simulink library "mfcm_misc_lib_v1"  (Simulink 6.1)
libraries: xbsIndex_r4 x81, mfcm_misc_lib_v1 x2, xbsCopyrightNotice_r4 x1, mfcm_mac_lib_v1 x1
settings Model: Creator=dandrews  LastModifiedBy=alexc

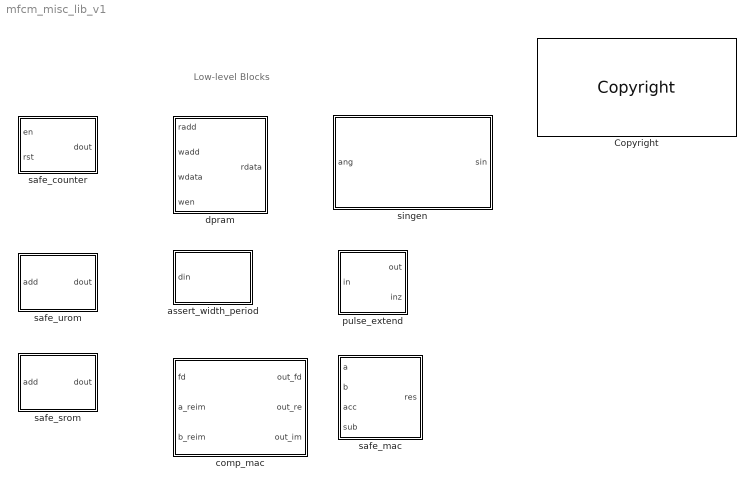
== system mfcm_misc_lib_v1 ==
  note: Low-level Blocks
  Copyright : xbsCopyrightNotice_r4/Copyright
  assert_width_period : Subsystem  mask{MIN_WIDTH=0, MAX_WIDTH=0, MIN_PERIOD=20, MAX_PERIOD=0}
      mask prompts: MIN_WIDTH "Minimum Pulse Width (0->none)"; MAX_WIDTH "Maximum Pulse Width (0->none)"; MIN_PERIOD "Minimum Pulse Period (0->none)"; MAX_PERIOD "Maximum Pulse Period (0->none)"
  comp_mac : Subsystem  mask{MULS=4, OUT_WIDTH=18, OUT_BINPT=16}
      mask prompts: MULS "Number of Multiplies"; OUT_WIDTH "Output Width"; OUT_BINPT "Output Binary Point"
      mask Display:
      | disp(sprintf('z^{%d}\n\n[z^{-(2*MULS+8)}]',-(2*MULS+8)),'texmode','on');
      | 
      | port_label('input',1,'fd');
      | port_label('input',2,'a_reim');
      | port_label('input',3,'b_reim');
      | 
      | port_label('output',1,'fd');
      | port_label('output',2,'re');
      | port_label('output',3,'im');
  dpram : Subsystem  mask{MEM_DEPTH=8192, MEM_INIT=0, MEM_MAXDEPTH=16}
      mask prompts: MEM_DEPTH "Memory Depth"; MEM_INIT "Memory Initialisation Vector"; MEM_MAXDEPTH "Maximum Distributed Memory Depth"
      mask Display:
      | disp('z^{-2}','texmode','on');
      | 
      | port_label('input',1,'radd');
      | port_label('input',2,'wadd');
      | port_label('input',3,'wdata');
      | port_label('input',4,'wen');
      | port_label('output',1,'rdata');
  pulse_extend : Subsystem  mask{WIDTH=1}
      mask prompts: WIDTH "Width of output pulse"
  safe_counter : Subsystem  mask{CNT_MAX=1}
      mask prompts: CNT_MAX "Count To Value"
      mask Display:
      | port_label('input' ,1,'en');
      | port_label('input' ,2,'rst');
      | port_label('output',1,'');
  safe_mac : Subsystem  mask{ACC_GROWTH=4, ACC_DEPTH=1}
      mask prompts: ACC_GROWTH "Accumulator Bit Width Growth"; ACC_DEPTH "Accumulator Pipeline Depth"
      mask Display:
      | disp('z^{-4}','texmode','on');
      | 
      | port_label('input',1,'a');
      | port_label('input',2,'b');
      | port_label('input',3,'acc');
      | port_label('input',4,'sub');
      | 
      | port_label('output',1,'res');
  safe_srom : Subsystem  mask{DEPTH=1, OUT_TYPE=1, OUT_WIDTH=8, OUT_BINPT=6, INIT=[1], LATENCY=1, MEM_MAXDEPTH=16}
      mask prompts: OUT_TYPE "Output Type (0->Boolean 1->Unsigned 2->Signed)"; OUT_WIDTH "Output Width"; OUT_BINPT "Output Binary Point"; INIT "Initialisation Vector"; MEM_MAXDEPTH "Maximum Distributed Memory Depth"
      mask Display:
      | disp(sprintf('z^{%d}',-LATENCY),'texmode','on');
      | port_label('input' ,1,'add');
      | port_label('output',1,'');
  safe_urom : Subsystem  mask{DEPTH=1, OUT_TYPE=1, OUT_WIDTH=8, OUT_BINPT=6, INIT=[1], LATENCY=1, MEM_MAXDEPTH=16}
      mask prompts: OUT_TYPE "Output Type (0->Boolean 1->Unsigned 2->Signed)"; OUT_WIDTH "Output Width"; OUT_BINPT "Output Binary Point"; INIT "Initialisation Vector"; MEM_MAXDEPTH "Maximum Distributed Memory Depth"
      mask Display:
      | disp(sprintf('z^{%d}',-LATENCY),'texmode','on');
      | port_label('input' ,1,'add');
      | port_label('output',1,'');
  singen : Subsystem  mask{N=8192, OUT_WIDTH=18, OUT_BINPT=17}
      mask prompts: N "Depth"; OUT_WIDTH "Output Width"; OUT_BINPT "Output Binary Point"
      mask Display:
      | disp('z^{-5}','texmode','on');
      | 
      | port_label('input',1,'ang');
      | 
      | port_label('output',1,'sin');

== system mfcm_misc_lib_v1/assert_width_period ==
  note: Wrap Mcode twice so we can use max() in MAX_CNT.
      | MCode interface does not support function calls.
  din : Inport  Port=1  LatchInput=off
  Terminator : Terminator
  x : Subsystem  mask{MIN_WIDTH=MIN_WIDTH, MAX_WIDTH=MAX_WIDTH, MIN_PERIOD=MIN_PERIOD, MAX_PERIOD=MAX_PERIOD, MAX_CNT=2^ceil(log2(max([MIN_WIDTH MAX_WIDTH MIN_PERIOD MAX_PERIOD])))}
  wires:
  x/1(fire) -> Terminator/1
  din/1 -> x/1(din)

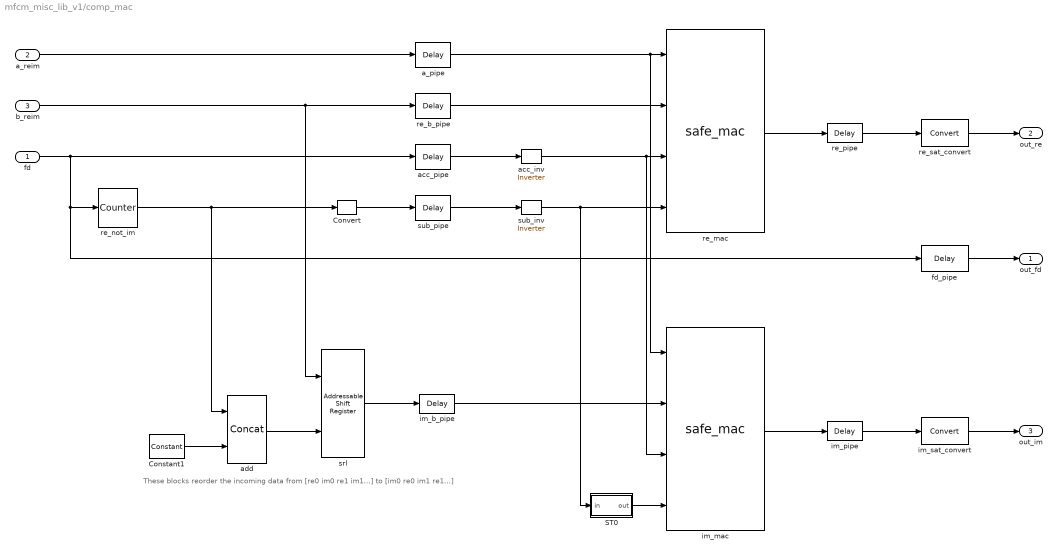
== system mfcm_misc_lib_v1/comp_mac ==
  note: These blocks reorder the incoming data from [re0 im0 re1 im1...] to [im0 re0 im1 re1...]
  fd : Inport  Port=1  LatchInput=off
  a_reim : Inport  Port=2  LatchInput=off
  b_reim : Inport  Port=3  LatchInput=off
  Constant1 : xbsIndex_r4/Constant  arith_type=Unsigned  const=0  n_bits=1  bin_pt=0  explicit_period=off  period=1  equ=P=C  opselect=C  inp2=PCIN>>17  opr=+  inp1=P  carry=CIN  dbl_ovrd=off  block_type=constant
      settings: block_version=VER_STRING_GOES_HERE
  Convert : xbsIndex_r4/Convert  arith_type=Boolean  n_bits=8  bin_pt=6  quantization=Truncate  overflow=Wrap  latency=0  dbl_ovrd=off  pipeline=off  block_type=convert
      settings: infoedit=The input is presented at the output after quantization and overflow effects.<P><P>Hardware notes: Additional hardware is used when rounding or saturation is selected and output width is less than the input width.  xl_area=[0, 0, 0, 0, 0, 0, 0]  block_version=VER_STRING_GOES_HERE
  ST0 : Subsystem
  a_pipe : xbsIndex_r4/Delay  en=off  latency=3  dbl_ovrd=off  reg_retiming=off  block_type=delay
      settings: infoedit="Delay line having  configurable length.<P><P>Hardware notes: A delay line is a chain, each link of which is an SRL16 followed by a flip-flop. If register retiming is enabled, the delay line is a chain of flip-flops."  xl_area=[0, 0, 0, 0, 0, 0, 0]  block_version=VER_STRING_GOES_HERE
  acc_inv : xbsIndex_r4/Inverter  en=off  latency=0  dbl_ovrd=off  block_type=inv
      settings: xl_area=[0, 0, 0, 0, 0, 0, 0]  block_version=VER_STRING_GOES_HERE
  acc_pipe : xbsIndex_r4/Delay  en=off  latency=3  dbl_ovrd=off  reg_retiming=off  block_type=delay
      settings: infoedit="Delay line having  configurable length.<P><P>Hardware notes: A delay line is a chain, each link of which is an SRL16 followed by a flip-flop. If register retiming is enabled, the delay line is a chain of flip-flops."  xl_area=[0, 0, 0, 0, 0, 0, 0]  block_version=VER_STRING_GOES_HERE
  add : xbsIndex_r4/Concat  num_inputs=2  dbl_ovrd=off  block_type=concat
      settings: block_version=VER_STRING_GOES_HERE
  fd_pipe : xbsIndex_r4/Delay  en=off  latency=2*MULS+3+4+2-1  dbl_ovrd=off  reg_retiming=off  block_type=delay
      settings: infoedit="Delay line having  configurable length.<P><P>Hardware notes: A delay line is a chain, each link of which is an SRL16 followed by a flip-flop. If register retiming is enabled, the delay line is a chain of flip-flops."  xl_area=[0, 0, 0, 0, 0, 0, 0]  block_version=VER_STRING_GOES_HERE
  im_b_pipe : xbsIndex_r4/Delay  en=off  latency=1  dbl_ovrd=off  reg_retiming=off  block_type=delay
      settings: infoedit="Delay line having  configurable length.<P><P>Hardware notes: A delay line is a chain, each link of which is an SRL16 followed by a flip-flop. If register retiming is enabled, the delay line is a chain of flip-flops."  xl_area=[0, 0, 0, 0, 0, 0, 0]  block_version=VER_STRING_GOES_HERE
  im_mac : mfcm_misc_lib_v1/safe_mac  ACC_GROWTH=ceil(log2(2*MULS))  ACC_DEPTH=1
  im_pipe : xbsIndex_r4/Delay  en=off  latency=1  dbl_ovrd=off  reg_retiming=off  block_type=delay
      settings: infoedit="Delay line having  configurable length.<P><P>Hardware notes: A delay line is a chain, each link of which is an SRL16 followed by a flip-flop. If register retiming is enabled, the delay line is a chain of flip-flops."  xl_area=[0, 0, 0, 0, 0, 0, 0]  block_version=VER_STRING_GOES_HERE
  im_sat_convert : xbsIndex_r4/Convert  arith_type="Signed  (2's comp)"  n_bits=OUT_WIDTH  bin_pt=OUT_BINPT  quantization=Truncate  overflow=Saturate  latency=1  dbl_ovrd=off  pipeline=off  block_type=convert
      settings: infoedit=The input is presented at the output after quantization and overflow effects.<P><P>Hardware notes: Additional hardware is used when rounding or saturation is selected and output width is less than the input width.  block_version=VER_STRING_GOES_HERE
  re_b_pipe : xbsIndex_r4/Delay  en=off  latency=3  dbl_ovrd=off  reg_retiming=off  block_type=delay
      settings: infoedit="Delay line having  configurable length.<P><P>Hardware notes: A delay line is a chain, each link of which is an SRL16 followed by a flip-flop. If register retiming is enabled, the delay line is a chain of flip-flops."  xl_area=[0, 0, 0, 0, 0, 0, 0]  block_version=VER_STRING_GOES_HERE
  re_mac : mfcm_misc_lib_v1/safe_mac  ACC_GROWTH=ceil(log2(2*MULS))  ACC_DEPTH=1
  re_not_im : xbsIndex_r4/Counter  cnt_type=Free Running  cnt_to=Inf  operation=Up  start_count=1  cnt_by_val=1  arith_type=Unsigned  n_bits=1  bin_pt=0  load_pin=off  rst=on  en=off  dbl_ovrd=off  explicit_period=off  period=1  block_type=counter
      settings: infoedit="Configurable up, down and up/down counter.<P><P>Hardware notes: Free running counters are the least expensive in hardware.  A count limited counter is implemented by combining a counter with a comparator."  xl_area=[0, 0, 0, 0, 0, 0, 0]  block_version=VER_STRING_GOES_HERE
  re_pipe : xbsIndex_r4/Delay  en=off  latency=1  dbl_ovrd=off  reg_retiming=off  block_type=delay
      settings: infoedit="Delay line having  configurable length.<P><P>Hardware notes: A delay line is a chain, each link of which is an SRL16 followed by a flip-flop. If register retiming is enabled, the delay line is a chain of flip-flops."  xl_area=[0, 0, 0, 0, 0, 0, 0]  block_version=VER_STRING_GOES_HERE
  re_sat_convert : xbsIndex_r4/Convert  arith_type="Signed  (2's comp)"  n_bits=OUT_WIDTH  bin_pt=OUT_BINPT  quantization=Truncate  overflow=Saturate  latency=1  dbl_ovrd=off  pipeline=off  block_type=convert
      settings: infoedit=The input is presented at the output after quantization and overflow effects.<P><P>Hardware notes: Additional hardware is used when rounding or saturation is selected and output width is less than the input width.  block_version=VER_STRING_GOES_HERE
  srl : xbsIndex_r4/Addressable Shift Register  infer_latency=on  depth=2  initVector=[0]  en=off  dbl_ovrd=off  use_behavioral_HDL=on  use_rpm=off  block_type=addrsr
      settings: infoedit="Delay of configurable length.  Any element in the delay line can be addressed and driven onto the output port.<P><P>Hardware notes: Implemented using SRL16s.  If a Virtex-II device is used, multiple SRLC16s are cascaded together."  xl_area=[0, 0, 0, 0, 0, 0, 0]  block_version=VER_STRING_GOES_HERE
  sub_inv : xbsIndex_r4/Inverter  en=off  latency=0  dbl_ovrd=off  block_type=inv
      settings: xl_area=[0, 0, 0, 0, 0, 0, 0]  block_version=VER_STRING_GOES_HERE
  sub_pipe : xbsIndex_r4/Delay  en=off  latency=2  dbl_ovrd=off  reg_retiming=off  block_type=delay
      settings: infoedit="Delay line having  configurable length.<P><P>Hardware notes: A delay line is a chain, each link of which is an SRL16 followed by a flip-flop. If register retiming is enabled, the delay line is a chain of flip-flops."  xl_area=[0, 0, 0, 0, 0, 0, 0]  block_version=VER_STRING_GOES_HERE
  out_fd : Outport
  out_re : Outport  Port=2
  out_im : Outport  Port=3
  wires:
  sub_pipe/1 -> sub_inv/1
  acc_pipe/1 -> acc_inv/1
  fd_pipe/1 -> out_fd/1
  a_reim/1 -> a_pipe/1
  re_mac/1 -> re_pipe/1
  b_reim/1 -> re_b_pipe/1, srl/1
  im_mac/1 -> im_pipe/1
  re_b_pipe/1 -> re_mac/2
  a_pipe/1 -> re_mac/1, im_mac/1
  fd/1 -> fd_pipe/1, re_not_im/1, acc_pipe/1
  im_sat_convert/1 -> out_im/1
  re_sat_convert/1 -> out_re/1
  ST0/1(out) -> im_mac/4
  im_b_pipe/1 -> im_mac/2
  re_not_im/1 -> add/1, Convert/1
  add/1 -> srl/2
  Constant1/1 -> add/2
  srl/1 -> im_b_pipe/1
  Convert/1 -> sub_pipe/1
  acc_inv/1 -> re_mac/3, im_mac/3
  sub_inv/1 -> ST0/1(in), re_mac/4
  re_pipe/1 -> re_sat_convert/1
  im_pipe/1 -> im_sat_convert/1

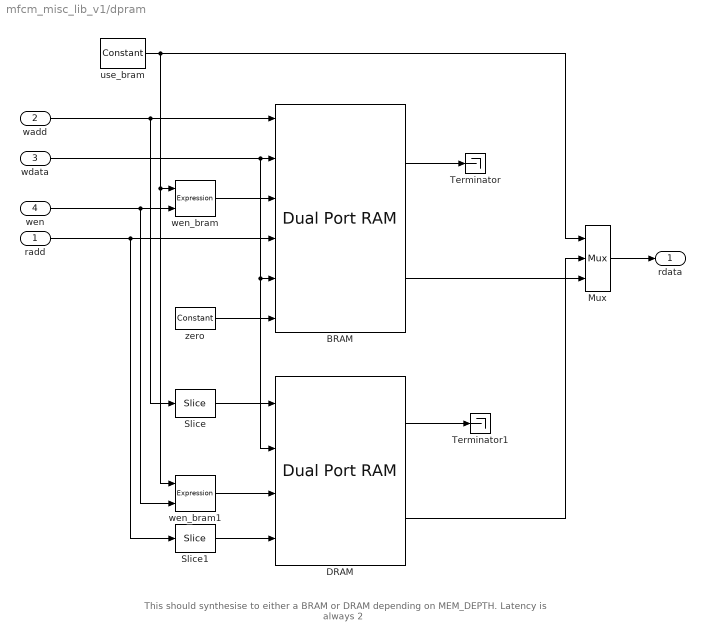
== system mfcm_misc_lib_v1/dpram ==
  note: This should synthesise to either a BRAM or DRAM depending on MEM_DEPTH.
      | Latency is always 2
  radd : Inport  Port=1  LatchInput=off
  wadd : Inport  Port=2  LatchInput=off
  wdata : Inport  Port=3  LatchInput=off
  wen : Inport  Port=4  LatchInput=off
  BRAM : xbsIndex_r4/Dual Port RAM  depth=MEM_DEPTH  initVector=MEM_INIT  distributed_mem=Block RAM  init_a=0  init_b=0  rst_a=off  rst_b=off  en_a=off  en_b=off  latency=2  write_mode_A=Read After Write  write_mode_B=Read After Write  dbl_ovrd=off  use_rpm=on  block_type=dpram
      settings: block_version=VER_STRING_GOES_HERE
  DRAM : xbsIndex_r4/Dual Port RAM  depth=min(MEM_DEPTH,MEM_MAXDEPTH)  initVector=MEM_INIT  distributed_mem=Distributed memory  init_a=0  init_b=0  rst_a=off  rst_b=off  en_a=off  en_b=off  latency=2  write_mode_A=Read After Write  write_mode_B=Read After Write  dbl_ovrd=off  use_rpm=on  block_type=dpram
      settings: block_version=VER_STRING_GOES_HERE
  Mux : xbsIndex_r4/Mux  inputs=2  en=off  latency=0  precision=Full  arith_type=Unsigned  n_bits=8  bin_pt=2  quantization=Truncate  overflow=Wrap  dbl_ovrd=off  block_type=mux
      settings: block_version=VER_STRING_GOES_HERE
  Slice : xbsIndex_r4/Slice  nbits=ceil(log2(min(MEM_DEPTH,MEM_MAXDEPTH)))  boolean_output=off  mode=Lower Bit Location + Width  bit1=0  base1=MSB of Input  bit0=0  base0=LSB of Input  dbl_ovrd=off  block_type=slice
      settings: infoedit="Extracts a given range of bits from each input sample and presents it at the output.  The output type is ordinarily unsigned with binary point at zero, but can be Boolean when the slice is one bit wide.<P><P>Hardware notes: In hardware this block costs nothing."  block_version=VER_STRING_GOES_HERE
  Slice1 : xbsIndex_r4/Slice  nbits=ceil(log2(min(MEM_DEPTH,MEM_MAXDEPTH)))  boolean_output=off  mode=Lower Bit Location + Width  bit1=0  base1=MSB of Input  bit0=0  base0=LSB of Input  dbl_ovrd=off  block_type=slice
      settings: infoedit="Extracts a given range of bits from each input sample and presents it at the output.  The output type is ordinarily unsigned with binary point at zero, but can be Boolean when the slice is one bit wide.<P><P>Hardware notes: In hardware this block costs nothing."  block_version=VER_STRING_GOES_HERE
  Terminator : Terminator
  Terminator1 : Terminator
  use_bram : xbsIndex_r4/Constant  arith_type=Boolean  const=double(MEM_DEPTH>MEM_MAXDEPTH)  n_bits=1  bin_pt=0  explicit_period=off  period=1  equ=P=C  opselect=C  inp2=PCIN>>17  opr=+  inp1=P  carry=CIN  dbl_ovrd=off  block_type=constant
      settings: block_version=VER_STRING_GOES_HERE
  wen_bram : xbsIndex_r4/Expression  expression=a & b  align_bp=on  en=off  latency=0  precision=Full  arith_type=Unsigned  n_bits=8  bin_pt=2  dbl_ovrd=off  block_type=expr
      settings: block_version=VER_STRING_GOES_HERE
  wen_bram1 : xbsIndex_r4/Expression  expression=~a & b  align_bp=on  en=off  latency=0  precision=Full  arith_type=Unsigned  n_bits=8  bin_pt=2  dbl_ovrd=off  block_type=expr
      settings: block_version=VER_STRING_GOES_HERE
  zero : xbsIndex_r4/Constant  arith_type=Boolean  const=0  n_bits=1  bin_pt=0  explicit_period=off  period=1  equ=P=C  opselect=C  inp2=PCIN>>17  opr=+  inp1=P  carry=CIN  dbl_ovrd=off  block_type=constant
      settings: block_version=VER_STRING_GOES_HERE
  rdata : Outport
  wires:
  Slice/1 -> DRAM/1
  wadd/1 -> BRAM/1, Slice/1
  wdata/1 -> BRAM/2, DRAM/2, BRAM/5
  wen_bram/1 -> BRAM/3
  use_bram/1 -> wen_bram/1, wen_bram1/1, Mux/1
  wen/1 -> wen_bram/2, wen_bram1/2
  wen_bram1/1 -> DRAM/3
  Slice1/1 -> DRAM/4
  radd/1 -> BRAM/4, Slice1/1
  zero/1 -> BRAM/6
  BRAM/1 -> Terminator/1
  DRAM/1 -> Terminator1/1
  BRAM/2 -> Mux/3
  DRAM/2 -> Mux/2
  Mux/1 -> rdata/1

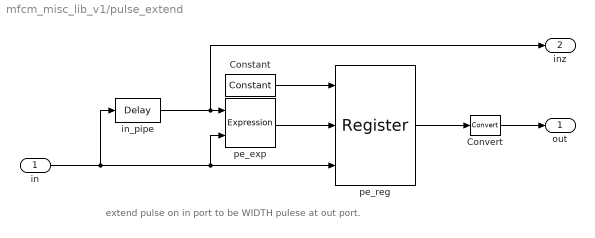
== system mfcm_misc_lib_v1/pulse_extend ==
  note: extend pulse on in port to be WIDTH pulese at out port.
  in : Inport  Port=1  LatchInput=off
  Constant : xbsIndex_r4/Constant  arith_type=Unsigned  const=1  n_bits=1  bin_pt=0  explicit_period=off  period=1  equ=P=C  opselect=C  inp2=PCIN>>17  opr=+  inp1=P  carry=CIN  dbl_ovrd=off  block_type=constant
      settings: block_version=VER_STRING_GOES_HERE
  Convert : xbsIndex_r4/Convert  arith_type=Boolean  n_bits=8  bin_pt=6  quantization=Truncate  overflow=Wrap  latency=0  dbl_ovrd=off  pipeline=off  block_type=convert
      settings: infoedit=The input is presented at the output after quantization and overflow effects.<P><P>Hardware notes: Additional hardware is used when rounding or saturation is selected and output width is less than the input width.  xl_area=[0, 0, 0, 0, 0, 0, 0]  block_version=VER_STRING_GOES_HERE
  in_pipe : xbsIndex_r4/Delay  en=off  latency=WIDTH  dbl_ovrd=off  reg_retiming=off  block_type=delay
      settings: infoedit="Delay line having  configurable length.<P><P>Hardware notes: A delay line is a chain, each link of which is an SRL16 followed by a flip-flop. If register retiming is enabled, the delay line is a chain of flip-flops."  xl_area=[0, 0, 0, 0, 0, 0, 0]  block_version=VER_STRING_GOES_HERE
  pe_exp : xbsIndex_r4/Expression  expression=a & ~b  align_bp=on  en=off  latency=0  precision=Full  arith_type=Unsigned  n_bits=8  bin_pt=2  dbl_ovrd=off  block_type=expr
      settings: xl_area=[0, 0, 0, 0, 0, 0, 0]  block_version=VER_STRING_GOES_HERE
  pe_reg : xbsIndex_r4/Register  init=0  rst=on  en=on  dbl_ovrd=off  block_type=register
      settings: xl_area=[0, 0, 0, 0, 0, 0, 0]  block_version=VER_STRING_GOES_HERE
  out : Outport
  inz : Outport  Port=2
  wires:
  in/1 -> pe_reg/3, pe_exp/2, in_pipe/1
  pe_exp/1 -> pe_reg/2
  in_pipe/1 -> pe_exp/1, inz/1
  Constant/1 -> pe_reg/1
  pe_reg/1 -> Convert/1
  Convert/1 -> out/1

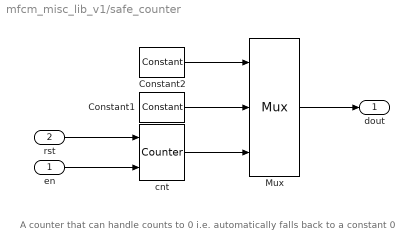
== system mfcm_misc_lib_v1/safe_counter ==
  note: A counter that can handle counts to 0
      | i.e. automatically falls back to a constant 0
  en : Inport  Port=1  LatchInput=off
  rst : Inport  Port=2  LatchInput=off
  Constant1 : xbsIndex_r4/Constant  arith_type=Unsigned  const=0  n_bits=1  bin_pt=0  explicit_period=off  period=1  equ=P=C  opselect=C  inp2=PCIN>>17  opr=+  inp1=P  carry=CIN  dbl_ovrd=off  block_type=constant
      settings: block_version=VER_STRING_GOES_HERE
  Constant2 : xbsIndex_r4/Constant  arith_type=Boolean  const=double(CNT_MAX>0)  n_bits=1  bin_pt=0  explicit_period=off  period=1  equ=P=C  opselect=C  inp2=PCIN>>17  opr=+  inp1=P  carry=CIN  dbl_ovrd=off  block_type=constant
      settings: block_version=VER_STRING_GOES_HERE
  Mux : xbsIndex_r4/Mux  inputs=2  en=off  latency=0  precision=Full  arith_type="Signed  (2's comp)"  n_bits=8  bin_pt=2  quantization=Truncate  overflow=Wrap  dbl_ovrd=off  block_type=mux
      settings: xl_area=[0, 0, 0, 0, 0, 0, 0]  block_version=VER_STRING_GOES_HERE
  cnt : xbsIndex_r4/Counter  cnt_type=Count Limited  cnt_to=max(CNT_MAX,1)  operation=Up  start_count=0  cnt_by_val=1  arith_type=Unsigned  n_bits=max(ceil(log2(CNT_MAX+1)),1)  bin_pt=0  load_pin=off  rst=on  en=on  dbl_ovrd=off  explicit_period=off  period=1  block_type=counter
      settings: infoedit="Configurable up, down and up/down counter.<P><P>Hardware notes: Free running counters are the least expensive in hardware.  A count limited counter is implemented by combining a counter with a comparator."  block_version=VER_STRING_GOES_HERE
  dout : Outport
  wires:
  Constant2/1 -> Mux/1
  Constant1/1 -> Mux/2
  cnt/1 -> Mux/3
  Mux/1 -> dout/1
  rst/1 -> cnt/1
  en/1 -> cnt/2

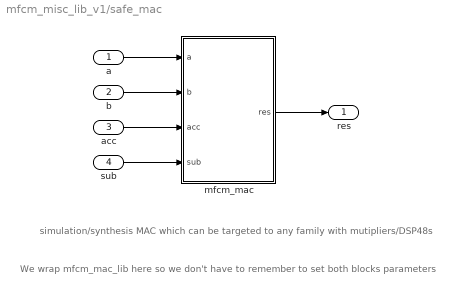
== system mfcm_misc_lib_v1/safe_mac ==
  note: simulation/synthesis MAC which can be targeted
      | to any family with mutipliers/DSP48s
  note: We wrap mfcm_mac_lib here so we don't have to
      | remember to set both blocks parameters
  a : Inport  Port=1  LatchInput=off
  b : Inport  Port=2  LatchInput=off
  acc : Inport  Port=3  LatchInput=off
  sub : Inport  Port=4  LatchInput=off
  mfcm_mac : Subsystem  Tag=configX  BlockChoice=mfcm_mac_sim
      link override mfcm_mac_sim: ACC_GROWTH=ACC_GROWTH  ACC_DEPTH=ACC_DEPTH
      link override mfcm_mac_syn: ACC_GROWTH=ACC_GROWTH  ACC_DEPTH=ACC_DEPTH
      settings: AttributesFormatString=%<BlockChoice>  TemplateBlock=mfcm_mac_lib_v1/mfcm_mac  MemberBlocks=mfcm_mac_sim,mfcm_mac_syn
  res : Outport
  wires:
  a/1 -> mfcm_mac/1(a)
  b/1 -> mfcm_mac/2(b)
  mfcm_mac/1(res) -> res/1
  acc/1 -> mfcm_mac/3(acc)
  sub/1 -> mfcm_mac/4(sub)

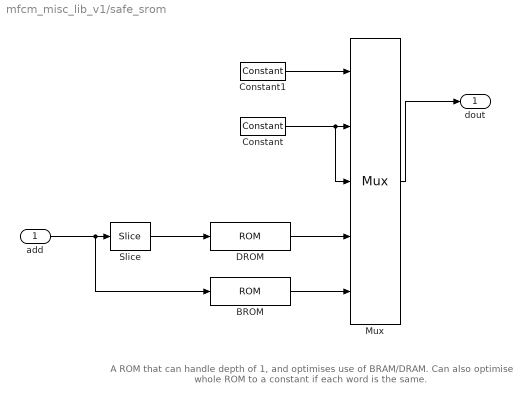
== system mfcm_misc_lib_v1/safe_srom ==
  note: A ROM that can handle depth of 1, and optimises use of BRAM/DRAM.
      | Can also optimise whole ROM to a constant if each word is the same.
  add : Inport  Port=1  LatchInput=off
  BROM : xbsIndex_r4/ROM  depth=max(DEPTH,2)  initVector=INIT  distributed_mem=Distributed memory  rst=off  init_reg=0  en=off  latency=LATENCY  arith_type="Signed  (2's comp)"  n_bits=OUT_WIDTH  bin_pt=OUT_BINPT  dbl_ovrd=off  use_rpm=off  block_type=sprom
      settings: xl_area=[0, 0, 0, 0, 0, 0, 0]  block_version=VER_STRING_GOES_HERE
  Constant : xbsIndex_r4/Constant  arith_type=Signed (2's comp)  const=min(INIT)  n_bits=OUT_WIDTH  bin_pt=OUT_BINPT  explicit_period=off  period=1  equ=P=C  opselect=C  inp2=PCIN>>17  opr=+  inp1=P  carry=CIN  dbl_ovrd=off  block_type=constant
      settings: block_version=VER_STRING_GOES_HERE
  Constant1 : xbsIndex_r4/Constant  arith_type=Unsigned  const=2*double(min(INIT)~=max(INIT))+double(DEPTH>MEM_MAXDEPTH)  n_bits=2  bin_pt=0  explicit_period=off  period=1  equ=P=C  opselect=C  inp2=PCIN>>17  opr=+  inp1=P  carry=CIN  dbl_ovrd=off  block_type=constant
      settings: block_version=VER_STRING_GOES_HERE
  DROM : xbsIndex_r4/ROM  depth=min(max(DEPTH,2),MEM_MAXDEPTH)  initVector=INIT  distributed_mem=Distributed memory  rst=off  init_reg=0  en=off  latency=LATENCY  arith_type="Signed  (2's comp)"  n_bits=OUT_WIDTH  bin_pt=OUT_BINPT  dbl_ovrd=off  use_rpm=off  block_type=sprom
      settings: xl_area=[0, 0, 0, 0, 0, 0, 0]  block_version=VER_STRING_GOES_HERE
  Mux : xbsIndex_r4/Mux  inputs=4  en=off  latency=0  precision=Full  arith_type="Signed  (2's comp)"  n_bits=8  bin_pt=2  quantization=Truncate  overflow=Wrap  dbl_ovrd=off  block_type=mux
      settings: xl_area=[0, 0, 0, 0, 0, 0, 0]  block_version=VER_STRING_GOES_HERE
  Slice : xbsIndex_r4/Slice  nbits=ceil(log2(min(max(DEPTH,2),MEM_MAXDEPTH)))  boolean_output=off  mode=Lower Bit Location + Width  bit1=0  base1=MSB of Input  bit0=0  base0=LSB of Input  dbl_ovrd=off  block_type=slice
      settings: infoedit="Extracts a given range of bits from each input sample and presents it at the output.  The output type is ordinarily unsigned with binary point at zero, but can be Boolean when the slice is one bit wide.<P><P>Hardware notes: In hardware this block costs nothing."  block_version=VER_STRING_GOES_HERE
  dout : Outport
  wires:
  Slice/1 -> DROM/1
  BROM/1 -> Mux/5
  DROM/1 -> Mux/4
  Constant/1 -> Mux/3, Mux/2
  add/1 -> BROM/1, Slice/1
  Mux/1 -> dout/1
  Constant1/1 -> Mux/1

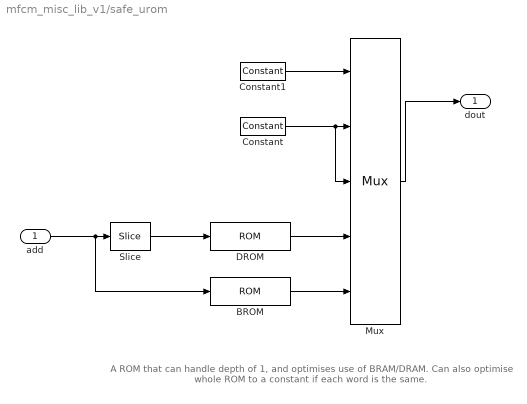
== system mfcm_misc_lib_v1/safe_urom ==
  note: A ROM that can handle depth of 1, and optimises use of BRAM/DRAM.
      | Can also optimise whole ROM to a constant if each word is the same.
  add : Inport  Port=1  LatchInput=off
  BROM : xbsIndex_r4/ROM  depth=max(DEPTH,2)  initVector=INIT  distributed_mem=Distributed memory  rst=off  init_reg=0  en=off  latency=LATENCY  arith_type=Unsigned  n_bits=OUT_WIDTH  bin_pt=OUT_BINPT  dbl_ovrd=off  use_rpm=off  block_type=sprom
      settings: xl_area=[0, 0, 0, 0, 0, 0, 0]  block_version=VER_STRING_GOES_HERE
  Constant : xbsIndex_r4/Constant  arith_type=Unsigned  const=min(INIT)  n_bits=OUT_WIDTH  bin_pt=OUT_BINPT  explicit_period=off  period=1  equ=P=C  opselect=C  inp2=PCIN>>17  opr=+  inp1=P  carry=CIN  dbl_ovrd=off  block_type=constant
      settings: block_version=VER_STRING_GOES_HERE
  Constant1 : xbsIndex_r4/Constant  arith_type=Unsigned  const=2*double(min(INIT)~=max(INIT))+double(DEPTH>MEM_MAXDEPTH)  n_bits=2  bin_pt=0  explicit_period=off  period=1  equ=P=C  opselect=C  inp2=PCIN>>17  opr=+  inp1=P  carry=CIN  dbl_ovrd=off  block_type=constant
      settings: block_version=VER_STRING_GOES_HERE
  DROM : xbsIndex_r4/ROM  depth=min(max(DEPTH,2),MEM_MAXDEPTH)  initVector=INIT  distributed_mem=Distributed memory  rst=off  init_reg=0  en=off  latency=LATENCY  arith_type=Unsigned  n_bits=OUT_WIDTH  bin_pt=OUT_BINPT  dbl_ovrd=off  use_rpm=off  block_type=sprom
      settings: xl_area=[0, 0, 0, 0, 0, 0, 0]  block_version=VER_STRING_GOES_HERE
  Mux : xbsIndex_r4/Mux  inputs=4  en=off  latency=0  precision=Full  arith_type="Signed  (2's comp)"  n_bits=8  bin_pt=2  quantization=Truncate  overflow=Wrap  dbl_ovrd=off  block_type=mux
      settings: xl_area=[0, 0, 0, 0, 0, 0, 0]  block_version=VER_STRING_GOES_HERE
  Slice : xbsIndex_r4/Slice  nbits=ceil(log2(min(max(DEPTH,2),MEM_MAXDEPTH)))  boolean_output=off  mode=Lower Bit Location + Width  bit1=0  base1=MSB of Input  bit0=0  base0=LSB of Input  dbl_ovrd=off  block_type=slice
      settings: infoedit="Extracts a given range of bits from each input sample and presents it at the output.  The output type is ordinarily unsigned with binary point at zero, but can be Boolean when the slice is one bit wide.<P><P>Hardware notes: In hardware this block costs nothing."  block_version=VER_STRING_GOES_HERE
  dout : Outport
  wires:
  Constant1/1 -> Mux/1
  Mux/1 -> dout/1
  add/1 -> Slice/1, BROM/1
  Constant/1 -> Mux/2, Mux/3
  DROM/1 -> Mux/4
  BROM/1 -> Mux/5
  Slice/1 -> DROM/1

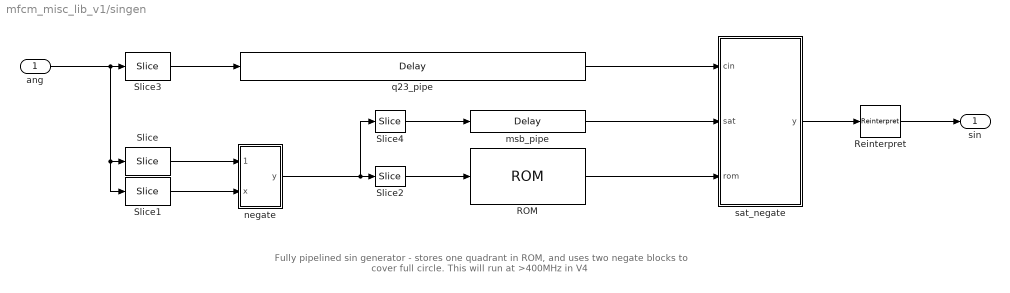
== system mfcm_misc_lib_v1/singen ==
  note: Fully pipelined sin generator - stores one quadrant in ROM, and uses two negate blocks to cover full circle.
      | This will run at >400MHz in V4
  ang : Inport  Port=1  LatchInput=off
  ROM : xbsIndex_r4/ROM  depth=N/4  initVector=min(round(sin([0:N/4-1]*2*pi/N)*2^OUT_BINPT),(2^OUT_WIDTH-1)-1)+floor(round(sin([0:N/4-1]*2*pi/N)*2^OUT_BINPT)/2^OUT_BINPT)*2^(OUT_WIDTH-1)*double((OUT_WIDTH-OUT_BINPT)<=1)  distributed_mem=Block RAM  rst=off  init_reg=0  en=off  latency=2  arith_type=Unsigned  n_bits=OUT_WIDTH  bin_pt=0  dbl_ovrd=off  use_rpm=off  block_type=sprom
      settings: xl_area=[0, 0, 0, 0, 0, 0, 0]  block_version=VER_STRING_GOES_HERE
  Reinterpret : xbsIndex_r4/Reinterpret  force_arith_type=on  arith_type="Signed  (2's comp)"  force_bin_pt=on  bin_pt=OUT_BINPT  block_type=cast
      settings: infoedit="Changes type of samples without altering their binary representation.<P><P>Hardware notes: In hardware this block costs nothing.<P><P>Example:  Suppose the input is 6 bits wide, signed, with 2 fractional bits, and the output is forced to unsigned with 0 fractional bits.  Then an input of -2.0 (1110.00 in binary 2's complement) becomes an output of 56 (111000 in binary)."  block_version=VER_STRING_GOES_HERE
  Slice : xbsIndex_r4/Slice  nbits=1  boolean_output=on  mode=Upper Bit Location + Width  bit1=-1  base1=MSB of Input  bit0=0  base0=LSB of Input  dbl_ovrd=off  block_type=slice
      settings: infoedit="Extracts a given range of bits from each input sample and presents it at the output.  The output type is ordinarily unsigned with binary point at zero, but can be Boolean when the slice is one bit wide.<P><P>Hardware notes: In hardware this block costs nothing."  block_version=VER_STRING_GOES_HERE
  Slice1 : xbsIndex_r4/Slice  nbits=log2(N)-2  boolean_output=off  mode=Lower Bit Location + Width  bit1=0  base1=MSB of Input  bit0=0  base0=LSB of Input  dbl_ovrd=off  block_type=slice
      settings: infoedit="Extracts a given range of bits from each input sample and presents it at the output.  The output type is ordinarily unsigned with binary point at zero, but can be Boolean when the slice is one bit wide.<P><P>Hardware notes: In hardware this block costs nothing."  block_version=VER_STRING_GOES_HERE
  Slice2 : xbsIndex_r4/Slice  nbits=log2(N)-2  boolean_output=off  mode=Lower Bit Location + Width  bit1=-1  base1=MSB of Input  bit0=0  base0=LSB of Input  dbl_ovrd=off  block_type=slice
      settings: infoedit="Extracts a given range of bits from each input sample and presents it at the output.  The output type is ordinarily unsigned with binary point at zero, but can be Boolean when the slice is one bit wide.<P><P>Hardware notes: In hardware this block costs nothing."  block_version=VER_STRING_GOES_HERE
  Slice3 : xbsIndex_r4/Slice  nbits=1  boolean_output=on  mode=Upper Bit Location + Width  bit1=0  base1=MSB of Input  bit0=0  base0=LSB of Input  dbl_ovrd=off  block_type=slice
      settings: infoedit="Extracts a given range of bits from each input sample and presents it at the output.  The output type is ordinarily unsigned with binary point at zero, but can be Boolean when the slice is one bit wide.<P><P>Hardware notes: In hardware this block costs nothing."  block_version=VER_STRING_GOES_HERE
  Slice4 : xbsIndex_r4/Slice  nbits=1  boolean_output=on  mode=Upper Bit Location + Width  bit1=0  base1=MSB of Input  bit0=0  base0=LSB of Input  dbl_ovrd=off  block_type=slice
      settings: infoedit="Extracts a given range of bits from each input sample and presents it at the output.  The output type is ordinarily unsigned with binary point at zero, but can be Boolean when the slice is one bit wide.<P><P>Hardware notes: In hardware this block costs nothing."  block_version=VER_STRING_GOES_HERE
  msb_pipe : xbsIndex_r4/Delay  en=off  latency=2  dbl_ovrd=off  reg_retiming=off  block_type=delay
      settings: infoedit="Delay line having  configurable length.<P><P>Hardware notes: A delay line is a chain, each link of which is an SRL16 followed by a flip-flop. If register retiming is enabled, the delay line is a chain of flip-flops."  xl_area=[0, 0, 0, 0, 0, 0, 0]  block_version=VER_STRING_GOES_HERE
  negate : Subsystem
  q23_pipe : xbsIndex_r4/Delay  en=off  latency=3  dbl_ovrd=off  reg_retiming=off  block_type=delay
      settings: infoedit="Delay line having  configurable length.<P><P>Hardware notes: A delay line is a chain, each link of which is an SRL16 followed by a flip-flop. If register retiming is enabled, the delay line is a chain of flip-flops."  xl_area=[0, 0, 0, 0, 0, 0, 0]  block_version=VER_STRING_GOES_HERE
  sat_negate : Subsystem
  sin : Outport
  wires:
  Slice3/1 -> q23_pipe/1
  ROM/1 -> sat_negate/3(rom)
  ang/1 -> Slice3/1, Slice1/1, Slice/1
  negate/1(y) -> Slice4/1, Slice2/1
  Slice2/1 -> ROM/1
  Slice4/1 -> msb_pipe/1
  msb_pipe/1 -> sat_negate/2(sat)
  sat_negate/1(y) -> Reinterpret/1
  Reinterpret/1 -> sin/1
  Slice/1 -> negate/1(negate)
  Slice1/1 -> negate/2(x)
  q23_pipe/1 -> sat_negate/1(cin)

== system mfcm_misc_lib_v1/assert_width_period/x ==
  din : Inport  Port=1  LatchInput=off
  x : xbsIndex_r4/MCode  mfname=mfcm_assert_width_period  explicit_period=off  period=1  dbl_ovrd=off  enable_debug=off  block_type=mcode  suppress_output=1  defparams={'MIN_WIDTH',MIN_WIDTH,'MAX_WIDTH',MAX_WIDTH,'MIN_PERIOD',MIN_PERIOD,'MAX_PERIOD',MAX_PERIOD,'MAX_CNT',16777215}  hide_port_list={}
      settings: block_version=8.1
  fire : Outport
  wires:
  din/1 -> x/1
  x/1 -> fire/1

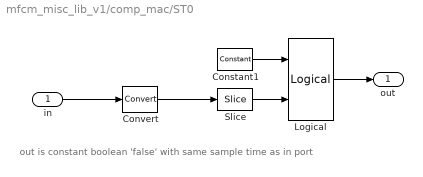
== system mfcm_misc_lib_v1/comp_mac/ST0 ==
  note: out is constant boolean 'false' with same
      | sample time as in port
  in : Inport  Port=1  LatchInput=off
  Constant1 : xbsIndex_r4/Constant  arith_type=Boolean  const=0  n_bits=1  bin_pt=0  explicit_period=off  period=1  equ=P=C  opselect=C  inp2=PCIN>>17  opr=+  inp1=P  carry=CIN  dbl_ovrd=off  block_type=constant
      settings: block_version=VER_STRING_GOES_HERE
  Convert : xbsIndex_r4/Convert  arith_type=Unsigned  n_bits=1  bin_pt=0  quantization=Truncate  overflow=Wrap  latency=0  dbl_ovrd=off  pipeline=off  block_type=convert
      settings: infoedit=The input is presented at the output after quantization and overflow effects.<P><P>Hardware notes: Additional hardware is used when rounding or saturation is selected and output width is less than the input width.  xl_area=[0, 0, 0, 0, 0, 0, 0]  block_version=VER_STRING_GOES_HERE
  Logical : xbsIndex_r4/Logical  logical_function=AND  inputs=2  en=off  latency=0  precision=Full  arith_type=Unsigned  n_bits=8  bin_pt=2  align_bp=on  dbl_ovrd=off  block_type=logical
      settings: xl_area=[0, 0, 0, 0, 0, 0, 0]  block_version=VER_STRING_GOES_HERE
  Slice : xbsIndex_r4/Slice  nbits=1  boolean_output=on  mode=Lower Bit Location + Width  bit1=0  base1=MSB of Input  bit0=0  base0=LSB of Input  dbl_ovrd=off  block_type=slice
      settings: infoedit="Extracts a given range of bits from each input sample and presents it at the output.  The output type is ordinarily unsigned with binary point at zero, but can be Boolean when the slice is one bit wide.<P><P>Hardware notes: In hardware this block costs nothing."  block_version=VER_STRING_GOES_HERE
  out : Outport
  wires:
  Constant1/1 -> Logical/1
  Convert/1 -> Slice/1
  in/1 -> Convert/1
  Logical/1 -> out/1
  Slice/1 -> Logical/2

== system mfcm_misc_lib_v1/safe_mac/mfcm_mac ==
  a : Inport  Port=1  LatchInput=off
  b : Inport  Port=2  LatchInput=off
  acc : Inport  Port=3  LatchInput=off
  sub : Inport  Port=4  LatchInput=off
  mfcm_mac_sim : mfcm_mac_lib_v1/mfcm_mac_sim  ACC_GROWTH=ACC_GROWTH  ACC_DEPTH=ACC_DEPTH
  res : Outport
  wires:
  a/1 -> mfcm_mac_sim/1
  b/1 -> mfcm_mac_sim/2
  acc/1 -> mfcm_mac_sim/3
  sub/1 -> mfcm_mac_sim/4
  mfcm_mac_sim/1 -> res/1

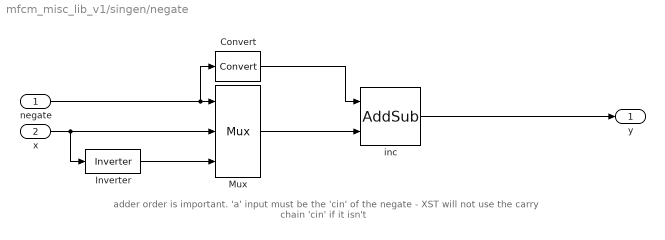
== system mfcm_misc_lib_v1/singen/negate ==
  note: adder order is important. 'a' input must be the 'cin' of the negate - XST will not use the carry chain 'cin' if it isn't
  negate : Inport  Port=1  LatchInput=off
  x : Inport  Port=2  LatchInput=off
  Convert : xbsIndex_r4/Convert  arith_type=Unsigned  n_bits=1  bin_pt=0  quantization=Truncate  overflow=Wrap  latency=0  dbl_ovrd=off  pipeline=off  block_type=convert
      settings: infoedit=The input is presented at the output after quantization and overflow effects.<P><P>Hardware notes: Additional hardware is used when rounding or saturation is selected and output width is less than the input width.  block_version=VER_STRING_GOES_HERE
  Inverter : xbsIndex_r4/Inverter  en=off  latency=0  dbl_ovrd=off  block_type=inv
      settings: block_version=VER_STRING_GOES_HERE
  Mux : xbsIndex_r4/Mux  inputs=2  en=off  latency=0  precision=Full  arith_type=Unsigned  n_bits=8  bin_pt=2  quantization=Truncate  overflow=Wrap  dbl_ovrd=off  block_type=mux
      settings: block_version=VER_STRING_GOES_HERE
  inc : xbsIndex_r4/AddSub  mode=Addition  use_carryin=off  use_carryout=off  en=off  latency=1  precision=Full  arith_type=Unsigned  n_bits=1  bin_pt=0  quantization=Truncate  overflow=Wrap  dbl_ovrd=off  use_behavioral_HDL=on  pipelined=off  use_rpm=on  block_type=addsub
      settings: block_version=VER_STRING_GOES_HERE
  y : Outport
  wires:
  Inverter/1 -> Mux/3
  x/1 -> Inverter/1, Mux/2
  negate/1 -> Mux/1, Convert/1
  inc/1 -> y/1
  Convert/1 -> inc/1
  Mux/1 -> inc/2

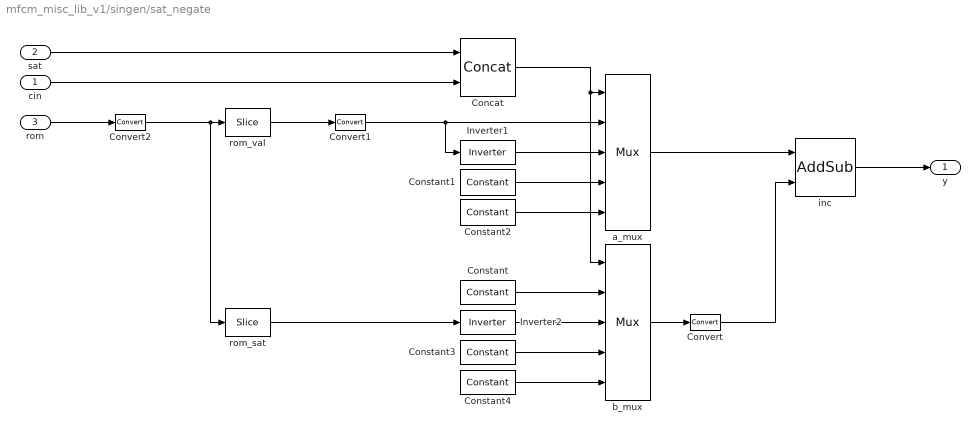
== system mfcm_misc_lib_v1/singen/sat_negate ==
  cin : Inport  Port=1  LatchInput=off
  sat : Inport  Port=2  LatchInput=off
  rom : Inport  Port=3  LatchInput=off
  Concat : xbsIndex_r4/Concat  num_inputs=2  dbl_ovrd=off  block_type=concat
      settings: block_version=VER_STRING_GOES_HERE
  Constant : xbsIndex_r4/Constant  arith_type=Boolean  const=0  n_bits=1  bin_pt=0  explicit_period=off  period=1  equ=P=C  opselect=C  inp2=PCIN>>17  opr=+  inp1=P  carry=CIN  dbl_ovrd=off  block_type=constant
      settings: block_version=VER_STRING_GOES_HERE
  Constant1 : xbsIndex_r4/Constant  arith_type=Unsigned  const=min(2^OUT_BINPT,2^(OUT_WIDTH-1)-1)  n_bits=OUT_WIDTH  bin_pt=0  explicit_period=off  period=1  equ=P=C  opselect=C  inp2=PCIN>>17  opr=+  inp1=P  carry=CIN  dbl_ovrd=off  block_type=constant
      settings: block_version=VER_STRING_GOES_HERE
  Constant2 : xbsIndex_r4/Constant  arith_type=Unsigned  const=2^OUT_WIDTH+max(-2^OUT_BINPT,-2^(OUT_WIDTH-1))-1  n_bits=OUT_WIDTH  bin_pt=0  explicit_period=off  period=1  equ=P=C  opselect=C  inp2=PCIN>>17  opr=+  inp1=P  carry=CIN  dbl_ovrd=off  block_type=constant
      settings: block_version=VER_STRING_GOES_HERE
  Constant3 : xbsIndex_r4/Constant  arith_type=Boolean  const=0  n_bits=1  bin_pt=0  explicit_period=off  period=1  equ=P=C  opselect=C  inp2=PCIN>>17  opr=+  inp1=P  carry=CIN  dbl_ovrd=off  block_type=constant
      settings: block_version=VER_STRING_GOES_HERE
  Constant4 : xbsIndex_r4/Constant  arith_type=Boolean  const=1  n_bits=1  bin_pt=0  explicit_period=off  period=1  equ=P=C  opselect=C  inp2=PCIN>>17  opr=+  inp1=P  carry=CIN  dbl_ovrd=off  block_type=constant
      settings: block_version=VER_STRING_GOES_HERE
  Convert : xbsIndex_r4/Convert  arith_type=Unsigned  n_bits=1  bin_pt=0  quantization=Truncate  overflow=Wrap  latency=0  dbl_ovrd=off  pipeline=off  block_type=convert
      settings: infoedit=The input is presented at the output after quantization and overflow effects.<P><P>Hardware notes: Additional hardware is used when rounding or saturation is selected and output width is less than the input width.  block_version=VER_STRING_GOES_HERE
  Convert1 : xbsIndex_r4/Convert  arith_type=Unsigned  n_bits=OUT_WIDTH  bin_pt=0  quantization=Truncate  overflow=Wrap  latency=0  dbl_ovrd=off  pipeline=off  block_type=convert
      settings: infoedit=The input is presented at the output after quantization and overflow effects.<P><P>Hardware notes: Additional hardware is used when rounding or saturation is selected and output width is less than the input width.  block_version=VER_STRING_GOES_HERE
  Convert2 : xbsIndex_r4/Convert  arith_type=Unsigned  n_bits=OUT_WIDTH+double((OUT_WIDTH-OUT_BINPT)>1)  bin_pt=0  quantization=Truncate  overflow=Wrap  latency=0  dbl_ovrd=off  pipeline=off  block_type=convert
      settings: infoedit=The input is presented at the output after quantization and overflow effects.<P><P>Hardware notes: Additional hardware is used when rounding or saturation is selected and output width is less than the input width.  block_version=VER_STRING_GOES_HERE
  Inverter1 : xbsIndex_r4/Inverter  en=off  latency=0  dbl_ovrd=off  block_type=inv
      settings: block_version=VER_STRING_GOES_HERE
  Inverter2 : xbsIndex_r4/Inverter  en=off  latency=0  dbl_ovrd=off  block_type=inv
      settings: block_version=VER_STRING_GOES_HERE
  a_mux : xbsIndex_r4/Mux  inputs=4  en=off  latency=1  precision=Full  arith_type=Unsigned  n_bits=8  bin_pt=2  quantization=Truncate  overflow=Wrap  dbl_ovrd=off  block_type=mux
      settings: block_version=VER_STRING_GOES_HERE
  b_mux : xbsIndex_r4/Mux  inputs=4  en=off  latency=1  precision=Full  arith_type=Unsigned  n_bits=8  bin_pt=2  quantization=Truncate  overflow=Wrap  dbl_ovrd=off  block_type=mux
      settings: block_version=VER_STRING_GOES_HERE
  inc : xbsIndex_r4/AddSub  mode=Addition  use_carryin=off  use_carryout=off  en=off  latency=1  precision=User Defined  arith_type=Unsigned  n_bits=OUT_WIDTH  bin_pt=0  quantization=Truncate  overflow=Wrap  dbl_ovrd=off  use_behavioral_HDL=on  pipelined=off  use_rpm=on  block_type=addsub
      settings: block_version=VER_STRING_GOES_HERE
  rom_sat : xbsIndex_r4/Slice  nbits=1  boolean_output=on  mode=Upper Bit Location + Width  bit1=0  base1=MSB of Input  bit0=0  base0=LSB of Input  dbl_ovrd=off  block_type=slice
      settings: infoedit="Extracts a given range of bits from each input sample and presents it at the output.  The output type is ordinarily unsigned with binary point at zero, but can be Boolean when the slice is one bit wide.<P><P>Hardware notes: In hardware this block costs nothing."  block_version=VER_STRING_GOES_HERE
  rom_val : xbsIndex_r4/Slice  nbits=OUT_WIDTH-double((OUT_WIDTH-OUT_BINPT)<=1)  boolean_output=off  mode=Lower Bit Location + Width  bit1=0  base1=MSB of Input  bit0=0  base0=LSB of Input  dbl_ovrd=off  block_type=slice
      settings: infoedit="Extracts a given range of bits from each input sample and presents it at the output.  The output type is ordinarily unsigned with binary point at zero, but can be Boolean when the slice is one bit wide.<P><P>Hardware notes: In hardware this block costs nothing."  block_version=VER_STRING_GOES_HERE
  y : Outport
  wires:
  Constant2/1 -> a_mux/5
  rom_sat/1 -> Inverter2/1
  Convert1/1 -> a_mux/2, Inverter1/1
  rom_val/1 -> Convert1/1
  Constant4/1 -> b_mux/5
  Constant3/1 -> b_mux/4
  Inverter2/1 -> b_mux/3
  Constant/1 -> b_mux/2
  Convert/1 -> inc/2
  b_mux/1 -> Convert/1
  Inverter1/1 -> a_mux/3
  cin/1 -> Concat/2
  Constant1/1 -> a_mux/4
  sat/1 -> Concat/1
  rom/1 -> Convert2/1
  inc/1 -> y/1
  a_mux/1 -> inc/1
  Convert2/1 -> rom_sat/1, rom_val/1
  Concat/1 -> a_mux/1, b_mux/1
